simulink model "p1"  (R2019b)
settings: Solver=VariableStepAuto  StartTime=0.0  StopTime=0.01  RelTol=1e-3
libraries: powerlib x20, powerlib_meascontrol x1
settings Model: Creator=sergiopiornoguemes  LastModifiedBy=deliaclar
settings DataIOCC: ReturnWorkspaceOutputs=off
settings DebuggingCC: ArithmeticOperatorsInVariantConditions=warning
settings SFSimCC: SimUseLocalCustomCode=off  CustomCodeUndefinedFunction=UseInterfaceOnly
settings RTWCC: RTWUseLocalCustomCode=off
settings CodeAppCC: StateflowObjectComments=on
settings SimscapeCC: SimscapeNormalizeSystem=off

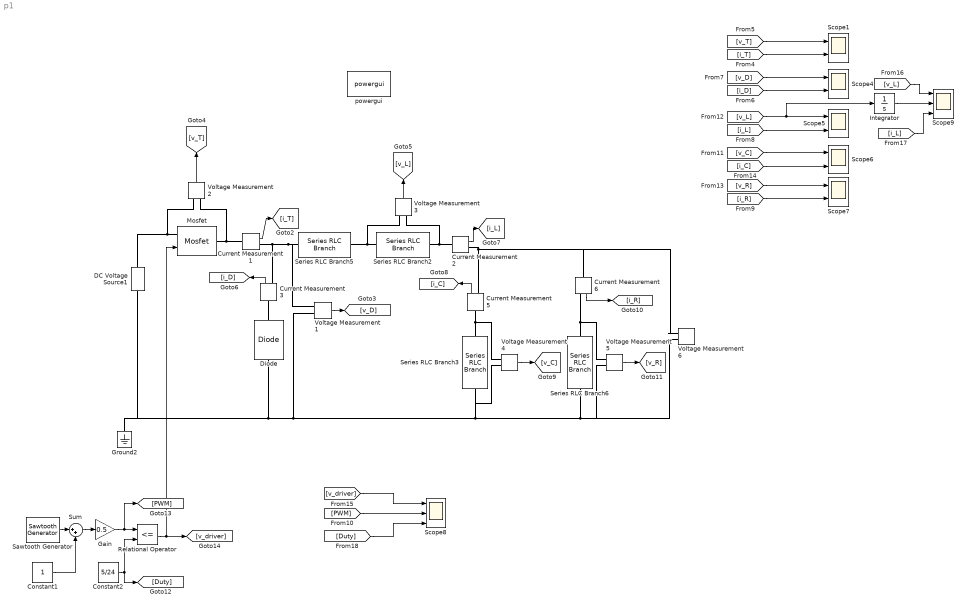
== system p1 ==
  Constant1 : Constant
  Constant2 : Constant  Value=5/24
  Current Measurement{1..3,5..6} (5 alike) : powerlib/Measurements/Current Measurement  PhasorSimulation=off  OutputType=Complex  PSBequivalent=0
      settings: SourceProductName=Simscape Electrical
  DC Voltage Source1 : powerlib/Electrical Sources/DC Voltage Source  Amplitude=24  Measurements=None
      settings: AttributesFormatString=Vs=%<Amplitude>  SourceProductName=Simscape Electrical
  Diode : powerlib/Power Electronics/Diode  Ron=0.001  Lon=0  Vf=0.8  IC=0  UseSnubber=off  Rs=500  Cs=250e-9  Measurements=off
      settings: SourceProductName=Simscape Electrical
  Gain : Gain  Gain=0.5
  Ground2 : powerlib/Elements/Ground  LConnTagsString=a
      settings: SourceProductName=Simscape Electrical
  Integrator : Integrator
  Mosfet : powerlib/Power Electronics/Mosfet  Ron=0.1  Lon=0  Rd=0.01  Vfd=0  IC=0  Rs=1e5  Cs=inf  Measurements=off
      settings: SourceProductName=Simscape Electrical
  Relational Operator : RelationalOperator  Operator=<=  OutDataTypeStr=boolean  RndMeth=Simplest
  Sawtooth Generator : powerlib_meascontrol/Pulse & Signal Generators/Sawtooth Generator  Freq=20e3  Phase=180  Ts=0
      settings: SourceProductName=Simscape Electrical
  Scope{1,4..7} (5 alike) : Scope  NumInputPorts=2
  Scope8 : Scope  NumInputPorts=3
  Scope9 : Scope  NumInputPorts=3
  Series RLC Branch2 : powerlib/Elements/Series RLC Branch  LConnTagsString=__new0  RConnTagsString=__new0  BranchType=L  Resistance=1  Inductance=1e-3  SetiL0=off  InitialCurrent=0  Capacitance=1e-6  Setx0=off  InitialVoltage=0  Measurements=None
      settings: SourceProductName=Simscape Electrical
  Series RLC Branch3 : powerlib/Elements/Series RLC Branch  LConnTagsString=__new0  RConnTagsString=__new0  BranchType=C  Resistance=1  Inductance=1e-3  SetiL0=off  InitialCurrent=0  Capacitance=22e-6  Setx0=off  InitialVoltage=0  Measurements=None
      settings: SourceProductName=Simscape Electrical
  Series RLC Branch5 : powerlib/Elements/Series RLC Branch  LConnTagsString=__new0  RConnTagsString=__new0  BranchType=R  Resistance=1  Inductance=1e-3  SetiL0=off  InitialCurrent=0  Capacitance=1e-6  Setx0=off  InitialVoltage=0  Measurements=None
      settings: SourceProductName=Simscape Electrical
  Series RLC Branch6 : powerlib/Elements/Series RLC Branch  LConnTagsString=__new0  RConnTagsString=__new0  BranchType=R  Resistance=6  Inductance=1e-3  SetiL0=off  InitialCurrent=0  Capacitance=1e-6  Setx0=off  InitialVoltage=0  Measurements=None
      settings: SourceProductName=Simscape Electrical
  Sum : Sum  Inputs=|++
  Voltage Measurement{1..6} (6 alike) : powerlib/Measurements/Voltage Measurement  PhasorSimulation=off  OutputType=Complex  PSBequivalent=0
      settings: SourceProductName=Simscape Electrical
  powergui : powerlib/powergui  Priority=1  SimulationMode=Continuous  SampleTime=50e-6  frequency=60  Iterations=50  frequencyindice=0  Pbase=100e6  ErrMax=1e-4  UnitsV=kV  UnitsW=MW  buscounter=0  FunctionMessages=off  echomessages=off  EnableUseOfTLC=off  CurrentSourceSwitches=off  DisableSnubberDevices=off  DisableRonSwitches=off  DisableVfSwitches=off  DisplayEquations=off  AutomaticDiscreteSolvers=off  SolverType=Tustin/Backward Euler (TBE)  Interpol=off  ExternalGateDelay=off  methode=off  Ts=10  x0status=blocks  SPID=off  SwTol=0  HookPort=off  NonlinearTolerance=1e-4  nMaxIteration=100  ContinueOnMaxIteration=off  RestoreLinks=warning  ResistiveCurrentMeasurement=off  Frange=[0:2:500]  Ylog=off  Xlog=on  ShowGrid=off  save=off  variable=ZData  structure=0  ZoomFFT=off  StartTime=0.0  cycles=1  DisplayStyle=1  fundamental=60  FreqAxis=off  MaxFrequency=1000  frequencyindicesteady=1  RmsSteady=1  display=off
      settings: SourceProductName=Simscape Electrical
  wires:
  Current Measurement1/1 -> [i_T]
  Voltage Measurement1/1 -> [v_D]
  Voltage Measurement2/1 -> [v_T]
  Voltage Measurement3/1 -> [v_L]
  Current Measurement3/1 -> [i_D]
  Current Measurement2/1 -> [i_L]
  Current Measurement5/1 -> [i_C]
  Voltage Measurement4/1 -> [v_C]
  Current Measurement6/1 -> [i_R]
  Voltage Measurement5/1 -> [v_R]
  Sawtooth Generator/1 -> Sum/1
  Constant1/1 -> Sum/2
  Sum/1 -> Gain/1
  Gain/1 -> [PWM], Relational Operator/1
  Constant2/1 -> [Duty], Relational Operator/2
  Relational Operator/1 -> Mosfet/1, [v_driver]
  [i_T] -> Scope1/2
  [v_T] -> Scope1/1
  [i_D] -> Scope4/2
  [v_D] -> Scope4/1
  [i_L] -> Scope5/2
  [v_L] -> Integrator/1, Scope5/1
  [i_C] -> Scope6/2
  [v_C] -> Scope6/1
  [i_R] -> Scope7/2
  [v_R] -> Scope7/1
  [PWM] -> Scope8/2
  [v_driver] -> Scope8/1
  Integrator/1 -> Scope9/2
  [v_L] -> Scope9/1
  [i_L] -> Scope9/3
  [Duty] -> Scope8/3
  connections:
  Series RLC Branch6/LConn1 -- Voltage Measurement5/LConn2 -- Voltage Measurement6/LConn2 -- Ground2/LConn1 -- DC Voltage Source1/LConn1 -- Diode/LConn1 -- Voltage Measurement1/LConn2 -- Voltage Measurement4/LConn2 -- Series RLC Branch3/LConn1
  Current Measurement1/RConn1 -- Current Measurement3/RConn1 -- Series RLC Branch5/RConn1 -- Voltage Measurement1/LConn1
  Series RLC Branch5/LConn1 -- Voltage Measurement3/LConn1 -- Series RLC Branch2/RConn1
  Current Measurement2/LConn1 -- Voltage Measurement3/LConn2 -- Series RLC Branch2/LConn1
  Mosfet/RConn1 -- Current Measurement1/LConn1 -- Voltage Measurement2/LConn2
  Voltage Measurement2/LConn1 -- DC Voltage Source1/RConn1 -- Mosfet/LConn1
  Current Measurement3/LConn1 -- Diode/RConn1
  Current Measurement2/RConn1 -- Voltage Measurement6/LConn1 -- Current Measurement6/LConn1 -- Current Measurement5/RConn1
  Current Measurement5/LConn1 -- Voltage Measurement4/LConn1 -- Series RLC Branch3/RConn1
  Voltage Measurement5/LConn1 -- Series RLC Branch6/RConn1 -- Current Measurement6/RConn1
